simulink model "EST"  (R2022b)
settings: Solver=FixedStepAuto  StartTime=0.0  StopTime=stopt  FixedStep=deltat/10  MaxStep=0.05  RelTol=1
InitFcn:
  | clear all;
  | close all;
  | clc;
  | 
  | % add the data and script directories
  | addpath('data','scripts');
  | 
  | % load the constants (units)
  | constants;
  | 
  | % load the simulation parameters
  | preprocessing;
StopFcn:
  | postprocessing;
model workspace (MAT data in the model file):
  TDeltaStorageInitial = Simulink.Parameter
  TDeltaStorageInitial.Value = 0
  TDeltaStorageInitial.DataType = 'auto'
  TDeltaStorageInitial.Complexity = 'real'
  TDeltaStorageInitial.Dimensions = [1 1]
  TStorageMax = Simulink.Parameter
  TStorageMax.Value = 10
  TStorageMax.DataType = 'auto'
  TStorageMax.Complexity = 'real'
  TStorageMax.Dimensions = [1 1]
  TStorageMin = Simulink.Parameter
  TStorageMin.Value = 0
  TStorageMin.DataType = 'auto'
  TStorageMin.Complexity = 'real'
  TStorageMin.Dimensions = [1 1]
values from neighbouring files (symbols this model uses):
  aDemandTransport = 0.02    [preprocessing.m]
  aExtraction = 0.11    [preprocessing.m]
  aNetInjection = 0.05    [preprocessing.m]
  areaOfTank = 6096*unit("m")*unit("m")    [preprocessing.m]
  bStorage = 1e-8/unit("s")    [preprocessing.m]
  e = 0.07    [preprocessing.m]
  efficiencyInverter = 0.97    [preprocessing.m]
  efficiencyTransformer = 0.99    [preprocessing.m]
  environmentalTemperature = 293*unit("K")    [preprocessing.m]
  EStorageInitial = 0.0*unit("kWh")    [preprocessing.m]
  EStorageMax = 450000*unit("kWh")    [preprocessing.m]
  EStorageMin = 0.0*unit("kWh")    [preprocessing.m]
  k = 0.04*unit("W")/unit("m")/unit("K")    [preprocessing.m]
  mass = 25837320*unit("kg")    [preprocessing.m]
  resistance = 0.00002373556*unit("ohm")    [preprocessing.m]
  sb = 5.670374419*10^-8*(     unit("W")/unit("m")/unit("m")/unit("K")/unit("K")/unit("K")/unit("K"))    [preprocessing.m]
  stringVoltage = 408*unit("V")    [preprocessing.m]
  x = 1*unit("m")    [preprocessing.m]
settings Model: Creator=joche  LastModifiedBy=20231162
settings DataIOCC: SaveFormat=Array  SaveOutput=off  ReturnWorkspaceOutputs=off
settings DebuggingCC: UnderSpecifiedDimensionMsg=warning
settings ModelReferenceCC: EnableRefExpFcnMdlSchedulingChecks=on

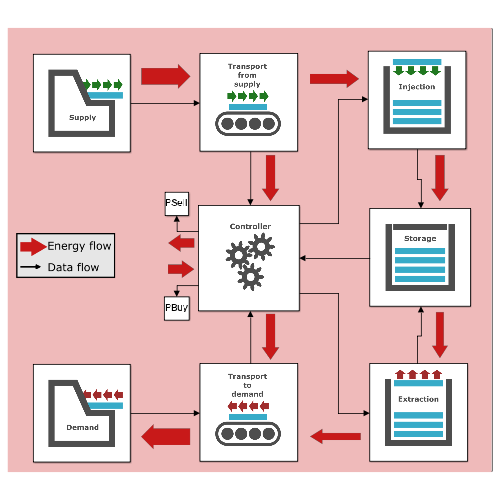
[thumbnail: Simulink's stored preview of the top-level diagram]
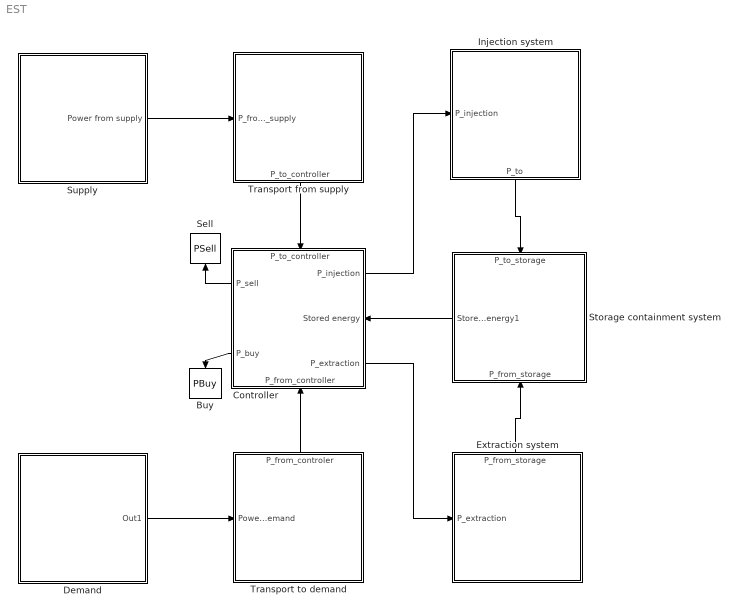
== system EST ==
  Buy : ToWorkspace  VariableName=PBuy  SampleTime=-1
  Controller : Subsystem
      settings: PortSchema="{\"entries\":[{\"content\":{\"sides\":[{\"content\":{\"connectorIds\":[\"Out3\",\"Out4\"]},\"type\":\"ConnectorPlacement.EquallySpacedRectSide\",\"uuid\":\"4daf33ce-c96a-4783-b5c4-228eed953e01\"},{\"content\":{\"connectorIds\":[\"Out1\",\"In3\",\"Out2\"],\"side\":\"RIGHT\"},\"type\":\"ConnectorPlacement.EquallySpacedRectSide\",\"uuid\":\"e9942e50-8467-4af8-b79b-80636cbc76e5\"},{\"content\":{\"connectorIds\":[\"In1\"],\"side\":\"TOP\"},\"type\":\"ConnectorPlacement.EquallySpacedRectSide\",\"uuid\":\"f315e931-d69b-4751-b712-f89c6c81baeb\"},{\"content\":{\"connectorIds\":[\"In2\"],\"side\":\"BOTTOM\"},\"type\":\"ConnectorPlacement.EquallySpacedRectSide\",\"uuid\":\"44715ee6-5cd5-4669-bcb9-5ed7c869bdb3\"}]},\"type\":\"ConnectorPlacement.EquallySpacedConnector\",\"uuid\":\"fff48899-944b-4064-b7d7-ecc12144fb48\"}],\"packageUris\":[\"http://schema.mathworks.com/mf0/Connector/R2020b\"],\"version\":\"1.0\"}"
      mask Display: image('$imagefile'); % Use "Edit Image" on toolstrip to change.
  Demand : Subsystem
      mask Display: image('$imagefile'); % Use "Edit Image" on toolstrip to change.
  Extraction system : Subsystem
      settings: PortSchema="{\"entries\":[{\"content\":{\"sides\":[{\"content\":{\"connectorIds\":[]},\"type\":\"ConnectorPlacement.EquallySpacedRectSide\",\"uuid\":\"05c5933d-55fc-4e06-853f-fc26d42905f9\"},{\"content\":{\"connectorIds\":[\"In1\"],\"side\":\"RIGHT\"},\"type\":\"ConnectorPlacement.EquallySpacedRectSide\",\"uuid\":\"327426c5-31d5-498b-a2bd-83e49353408c\"},{\"content\":{\"connectorIds\":[],\"side\":\"TOP\"},\"type\":\"ConnectorPlacement.EquallySpacedRectSide\",\"uuid\":\"55306cf3-a3de-4385-a5ae-b8600ecdd5a2\"},{\"content\":{\"connectorIds\":[\"Out1\"],\"side\":\"BOTTOM\"},\"type\":\"ConnectorPlacement.EquallySpacedRectSide\",\"uuid\":\"08fcc9c3-40d3-4ac6-b914-dfeef6039ffb\"}]},\"type\":\"ConnectorPlacement.EquallySpacedConnector\",\"uuid\":\"cb35d5ba-e8c6-462c-b7b2-fe8356d4b0a1\"}],\"packageUris\":[\"http://schema.mathworks.com/mf0/Connector/R2020b\"],\"version\":\"1.0\"}"
      mask Display: image('$imagefile'); % Use "Edit Image" on toolstrip to change.
  Injection system : Subsystem
      settings: PortSchema="{\"entries\":[{\"content\":{\"sides\":[{\"content\":{\"connectorIds\":[]},\"type\":\"ConnectorPlacement.EquallySpacedRectSide\",\"uuid\":\"05c5933d-55fc-4e06-853f-fc26d42905f9\"},{\"content\":{\"connectorIds\":[\"In1\"],\"side\":\"RIGHT\"},\"type\":\"ConnectorPlacement.EquallySpacedRectSide\",\"uuid\":\"327426c5-31d5-498b-a2bd-83e49353408c\"},{\"content\":{\"connectorIds\":[\"Out1\"],\"side\":\"TOP\"},\"type\":\"ConnectorPlacement.EquallySpacedRectSide\",\"uuid\":\"55306cf3-a3de-4385-a5ae-b8600ecdd5a2\"},{\"content\":{\"connectorIds\":[],\"side\":\"BOTTOM\"},\"type\":\"ConnectorPlacement.EquallySpacedRectSide\",\"uuid\":\"08fcc9c3-40d3-4ac6-b914-dfeef6039ffb\"}]},\"type\":\"ConnectorPlacement.EquallySpacedConnector\",\"uuid\":\"cb35d5ba-e8c6-462c-b7b2-fe8356d4b0a1\"}],\"packageUris\":[\"http://schema.mathworks.com/mf0/Connector/R2020b\"],\"version\":\"1.0\"}"
      mask Display: image('$imagefile'); % Use "Edit Image" on toolstrip to change.
  Sell : ToWorkspace  VariableName=PSell  SampleTime=-1
  Storage containment system : Subsystem
      settings: PortSchema="{\"entries\":[{\"content\":{\"sides\":[{\"content\":{\"connectorIds\":[\"Out1\"]},\"type\":\"ConnectorPlacement.EquallySpacedRectSide\",\"uuid\":\"0ba48424-33b9-4934-970f-64fe5d8b070e\"},{\"content\":{\"connectorIds\":[],\"side\":\"RIGHT\"},\"type\":\"ConnectorPlacement.EquallySpacedRectSide\",\"uuid\":\"9cde340f-8f39-4499-9a12-5e1623737660\"},{\"content\":{\"connectorIds\":[\"In1\"],\"side\":\"TOP\"},\"type\":\"ConnectorPlacement.EquallySpacedRectSide\",\"uuid\":\"2af8db04-7fd0-4902-8637-8dc00edb4598\"},{\"content\":{\"connectorIds\":[\"In2\"],\"side\":\"BOTTOM\"},\"type\":\"ConnectorPlacement.EquallySpacedRectSide\",\"uuid\":\"e21ea806-d777-41a3-a53f-556fae66854b\"}]},\"type\":\"ConnectorPlacement.EquallySpacedConnector\",\"uuid\":\"4e2ddb36-4db3-4ab4-858b-ebb8ccefeb1f\"}],\"packageUris\":[\"http://schema.mathworks.com/mf0/Connector/R2020b\"],\"version\":\"1.0\"}"
      mask Display: image('$imagefile'); % Use "Edit Image" on toolstrip to change.
  Supply : Subsystem
      mask Display: image('$imagefile'); % Use "Edit Image" on toolstrip to change.
  Transport from supply : Subsystem
      settings: PortSchema="{\"entries\":[{\"content\":{\"sides\":[{\"content\":{\"connectorIds\":[\"In1\"]},\"type\":\"ConnectorPlacement.EquallySpacedRectSide\",\"uuid\":\"31329006-3d36-4d93-9c44-7503a515d397\"},{\"content\":{\"connectorIds\":[],\"side\":\"RIGHT\"},\"type\":\"ConnectorPlacement.EquallySpacedRectSide\",\"uuid\":\"aba139c7-f9b6-4881-a56b-a4cbbedacd88\"},{\"content\":{\"connectorIds\":[],\"side\":\"TOP\"},\"type\":\"ConnectorPlacement.EquallySpacedRectSide\",\"uuid\":\"e683eb73-7a35-4160-9c39-da83856a6278\"},{\"content\":{\"connectorIds\":[\"Out1\"],\"side\":\"BOTTOM\"},\"type\":\"ConnectorPlacement.EquallySpacedRectSide\",\"uuid\":\"1170dd18-447c-437f-9043-6812c2877331\"}]},\"type\":\"ConnectorPlacement.EquallySpacedConnector\",\"uuid\":\"804af608-1d70-444f-af69-e05f19bf98f3\"}],\"packageUris\":[\"http://schema.mathworks.com/mf0/Connector/R2020b\"],\"version\":\"1.0\"}"
      mask Display: image('$imagefile'); % Use "Edit Image" on toolstrip to change.
  Transport to demand : Subsystem
      settings: PortSchema="{\"entries\":[{\"content\":{\"sides\":[{\"content\":{\"connectorIds\":[\"In1\"]},\"type\":\"ConnectorPlacement.EquallySpacedRectSide\",\"uuid\":\"31329006-3d36-4d93-9c44-7503a515d397\"},{\"content\":{\"connectorIds\":[],\"side\":\"RIGHT\"},\"type\":\"ConnectorPlacement.EquallySpacedRectSide\",\"uuid\":\"aba139c7-f9b6-4881-a56b-a4cbbedacd88\"},{\"content\":{\"connectorIds\":[\"Out1\"],\"side\":\"TOP\"},\"type\":\"ConnectorPlacement.EquallySpacedRectSide\",\"uuid\":\"e683eb73-7a35-4160-9c39-da83856a6278\"},{\"content\":{\"connectorIds\":[],\"side\":\"BOTTOM\"},\"type\":\"ConnectorPlacement.EquallySpacedRectSide\",\"uuid\":\"c378138f-7233-4483-870c-40a69b3495ee\"}]},\"type\":\"ConnectorPlacement.EquallySpacedConnector\",\"uuid\":\"804af608-1d70-444f-af69-e05f19bf98f3\"}],\"packageUris\":[\"http://schema.mathworks.com/mf0/Connector/R2020b\"],\"version\":\"1.0\"}"
      mask Display: image('$imagefile'); % Use "Edit Image" on toolstrip to change.
  wires:
  Supply/1(Power from supply) -> Transport from supply/1(P_from_supply)
  Transport from supply/1(P_to_controller) -> Controller/1(P_to_controller)
  Transport to demand/1(P_from_controler) -> Controller/2(P_from_controller)
  Demand/1(Out1) -> Transport to demand/1(Power to demand)
  Controller/3(P_sell) -> Sell/1
  Controller/2(P_extraction) -> Extraction system/1(P_extraction)
  Injection system/1(P_to) -> Storage containment system/1(P_to_storage)
  Extraction system/1(P_from_storage) -> Storage containment system/2(P_from_storage)
  Storage containment system/1(Stored energy1) -> Controller/3(Stored energy)
  Controller/1(P_injection) -> Injection system/1(P_injection)
  Controller/4(P_buy) -> Buy/1

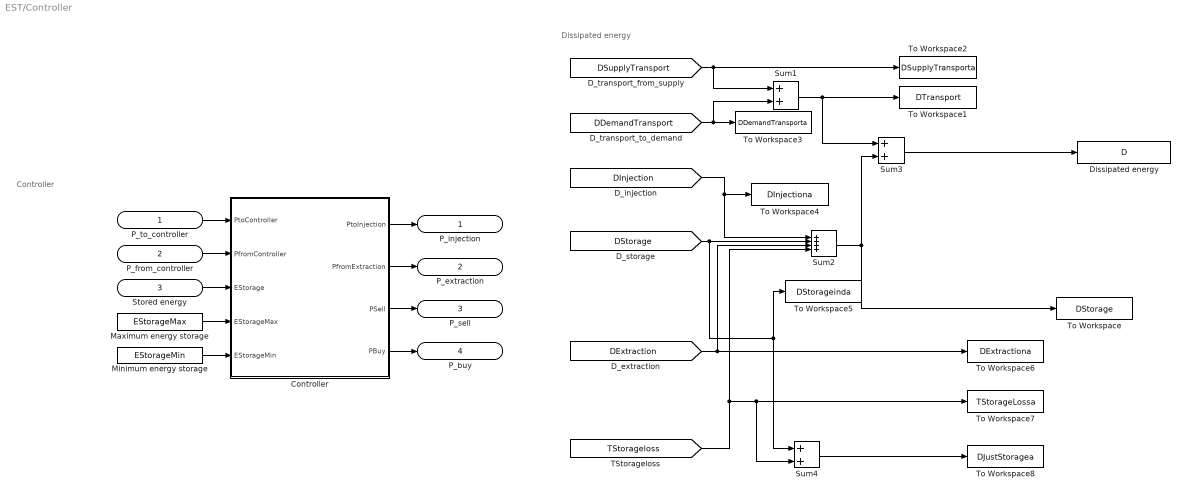
== system EST/Controller ==
  note: Dissipated energy
  note: Controller
  P_to_controller : Inport
  P_from_controller : Inport  Port=2
  Stored energy : Inport  Port=3
  Controller : MATLAB Function  TreatAsAtomicUnit=on
  Dissipated energy : ToWorkspace  VariableName=D  SampleTime=-1
  Maximum energy storage : Constant  Value=EStorageMax
  Minimum energy storage : Constant  Value=EStorageMin
  Sum1 : Sum
  Sum2 : Sum  Inputs=++++
  Sum3 : Sum
  Sum4 : Sum
  To Workspace : ToWorkspace  VariableName=DStorage  SampleTime=-1
  To Workspace1 : ToWorkspace  VariableName=DTransport  SampleTime=-1
  To Workspace2 : ToWorkspace  VariableName=DSupplyTransporta  SampleTime=-1
  To Workspace3 : ToWorkspace  VariableName=DDemandTransporta  SampleTime=-1
  To Workspace4 : ToWorkspace  VariableName=DInjectiona  SampleTime=-1
  To Workspace5 : ToWorkspace  VariableName=DStorageinda  SampleTime=-1
  To Workspace6 : ToWorkspace  VariableName=DExtractiona  SampleTime=-1
  To Workspace7 : ToWorkspace  VariableName=TStorageLossa  SampleTime=-1
  To Workspace8 : ToWorkspace  VariableName=DJustStoragea  SampleTime=-1
  P_injection : Outport
  P_extraction : Outport  Port=2
  P_sell : Outport  Port=3
  P_buy : Outport  Port=4
  wires:
  P_from_controller/1 -> Controller/2(PfromController)
  Controller/2(PfromExtraction) -> P_extraction/1
  Controller/3(PSell) -> P_sell/1
  Controller/4(PBuy) -> P_buy/1
  Minimum energy storage/1 -> Controller/5(EStorageMin)
  Maximum energy storage/1 -> Controller/4(EStorageMax)
  P_to_controller/1 -> Controller/1(PtoController)
  Controller/1(PtoInjection) -> P_injection/1
  Stored energy/1 -> Controller/3(EStorage)
  [DDemandTransport] -> Sum1/2, To Workspace3/1
  [DSupplyTransport] -> Sum1/1, To Workspace2/1
  [DInjection] -> Sum2/1, To Workspace4/1
  [DStorage] -> Sum2/2, Sum4/1, To Workspace5/1
  [DExtraction] -> Sum2/3, To Workspace6/1
  Sum2/1 -> To Workspace/1, Sum3/2
  Sum1/1 -> Sum3/1, To Workspace1/1
  Sum3/1 -> Dissipated energy/1
  [TStorageloss] -> Sum2/4, Sum4/2, To Workspace7/1
  Sum4/1 -> To Workspace8/1

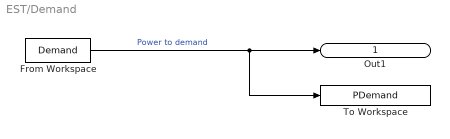
== system EST/Demand ==
  From Workspace : FromWorkspace  VariableName=Demand  OutputAfterFinalValue=Setting to zero
  To Workspace : ToWorkspace  VariableName=PDemand  SampleTime=-1
  Out1 : Outport
  wires:
  From Workspace/1 -> To Workspace/1, Out1/1  "Power to demand"

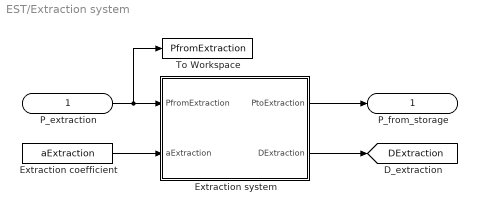
== system EST/Extraction system ==
  P_extraction : Inport
  Extraction coefficient : Constant  Value=aExtraction
  Extraction system : MATLAB Function  TreatAsAtomicUnit=on
  To Workspace : ToWorkspace  VariableName=PfromExtraction  SampleTime=-1
  P_from_storage : Outport
  tag scope: DExtraction=global
  wires:
  P_extraction/1 -> To Workspace/1, Extraction system/1(PfromExtraction)
  Extraction system/1(PtoExtraction) -> P_from_storage/1
  Extraction coefficient/1 -> Extraction system/2(aExtraction)
  Extraction system/2(DExtraction) -> [DExtraction]

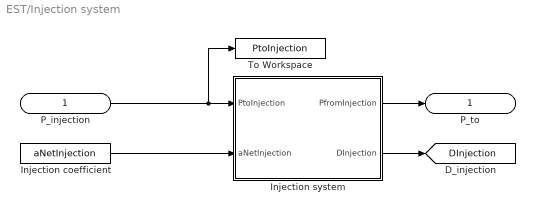
== system EST/Injection system ==
  P_injection : Inport
  Injection coefficient : Constant  Value=aNetInjection
  Injection system : MATLAB Function  TreatAsAtomicUnit=on
  To Workspace : ToWorkspace  VariableName=PtoInjection  SampleTime=-1
  P_to : Outport
  tag scope: DInjection=global
  wires:
  P_injection/1 -> To Workspace/1, Injection system/1(PtoInjection)
  Injection system/1(PfromInjection) -> P_to/1
  Injection coefficient/1 -> Injection system/2(aNetInjection)
  Injection system/2(DInjection) -> [DInjection]

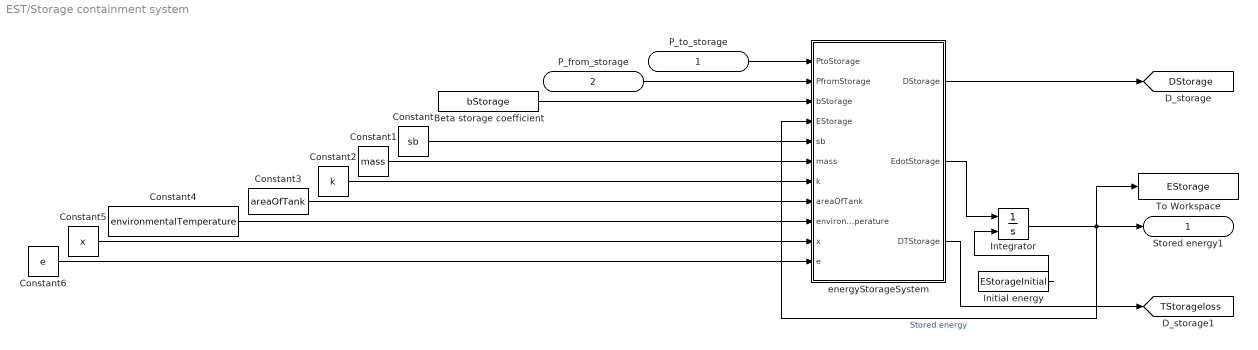
== system EST/Storage containment system ==
  P_to_storage : Inport
  P_from_storage : Inport  Port=2
  Beta storage coefficient : Constant  Value=bStorage
  Constant : Constant  Value=sb
  Constant1 : Constant  Value=mass
  Constant2 : Constant  Value=k
  Constant3 : Constant  Value=areaOfTank
  Constant4 : Constant  Value=environmentalTemperature
  Constant5 : Constant  Value=x
  Constant6 : Constant  Value=e
  Initial energy : Constant  Value=EStorageInitial
  Integrator : Integrator  InitialConditionSource=external
  To Workspace : ToWorkspace  VariableName=EStorage  SampleTime=-1
  energyStorageSystem : MATLAB Function  TreatAsAtomicUnit=on
  Stored energy1 : Outport
  tag scope: DStorage=global, TStorageloss=global
  wires:
  Initial energy/1 -> Integrator/2
  Integrator/1 -> To Workspace/1, energyStorageSystem/4(EStorage), Stored energy1/1  "Stored energy"
  energyStorageSystem/1(DStorage) -> [DStorage]
  Beta storage coefficient/1 -> energyStorageSystem/3(bStorage)
  energyStorageSystem/2(EdotStorage) -> Integrator/1
  P_to_storage/1 -> energyStorageSystem/1(PtoStorage)
  P_from_storage/1 -> energyStorageSystem/2(PfromStorage)
  energyStorageSystem/3(DTStorage) -> [TStorageloss]
  Constant/1 -> energyStorageSystem/5(sb)
  Constant1/1 -> energyStorageSystem/6(mass)
  Constant2/1 -> energyStorageSystem/7(k)
  Constant3/1 -> energyStorageSystem/8(areaOfTank)
  Constant4/1 -> energyStorageSystem/9(environmentalTemperature)
  Constant5/1 -> energyStorageSystem/10(x)
  Constant6/1 -> energyStorageSystem/11(e)

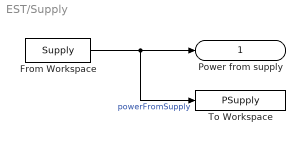
== system EST/Supply ==
  From Workspace : FromWorkspace  VariableName=Supply  OutputAfterFinalValue=Setting to zero
  To Workspace : ToWorkspace  VariableName=PSupply  SampleTime=-1
  Power from supply : Outport
  wires:
  From Workspace/1 -> To Workspace/1, Power from supply/1  "powerFromSupply"

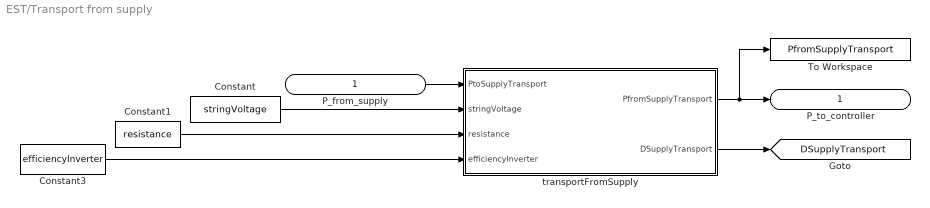
== system EST/Transport from supply ==
  P_from_supply : Inport
  " transportFromSupply" : MATLAB Function  TreatAsAtomicUnit=on
  Constant : Constant  Value=stringVoltage
  Constant1 : Constant  Value=resistance
  Constant3 : Constant  Value=efficiencyInverter
  To Workspace : ToWorkspace  VariableName=PfromSupplyTransport  SampleTime=-1
  P_to_controller : Outport
  tag scope: DSupplyTransport=global
  wires:
  P_from_supply/1 -> " transportFromSupply"/1(PtoSupplyTransport)
  " transportFromSupply"/1(PfromSupplyTransport) -> To Workspace/1, P_to_controller/1
  " transportFromSupply"/2(DSupplyTransport) -> [DSupplyTransport]
  Constant/1 -> " transportFromSupply"/2(stringVoltage)
  Constant1/1 -> " transportFromSupply"/3(resistance)
  Constant3/1 -> " transportFromSupply"/4(efficiencyInverter)

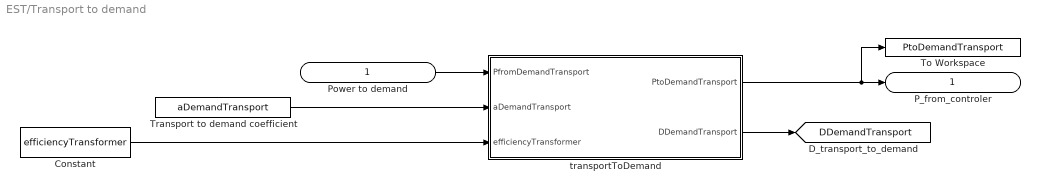
== system EST/Transport to demand ==
  Power to demand : Inport
  Constant : Constant  Value=efficiencyTransformer
  To Workspace : ToWorkspace  VariableName=PtoDemandTransport  SampleTime=-1
  Transport to demand coefficient : Constant  Value=aDemandTransport
  transportToDemand : MATLAB Function  TreatAsAtomicUnit=on
  P_from_controler : Outport
  tag scope: DDemandTransport=global
  wires:
  Transport to demand coefficient/1 -> transportToDemand/2(aDemandTransport)
  transportToDemand/2(DDemandTransport) -> [DDemandTransport]
  transportToDemand/1(PtoDemandTransport) -> To Workspace/1, P_from_controler/1
  Power to demand/1 -> transportToDemand/1(PfromDemandTransport)
  Constant/1 -> transportToDemand/3(efficiencyTransformer)

== matlab function EST/Injection system/Injection system ==
  data: PtoInjection input; PfromInjection output; aNetInjection input; DInjection output
function [PfromInjection, DInjection] = injection(PtoInjection, aNetInjection ...
    )
    %
    % This function calculates the power signal and coreresponding loss 
    % after the injection. The returned power signal goes to the air energy
    % storage as well as the thermal storage.
    %
    % Parameters:
    %   PtoInjection: A double with the power signals coming from the
    %                 supply required by the controller with the same array 
    %                 dimensions as tout.
    %   aInjection:   A double of size 1x1 which is the loss coeficient
    %                 during injection.
    %
    % Returns:
    %   double: PfromInjection, the power signal with the same
    %           array dimensions as PtoInjection. Goes to the storage.
    %   double: DInjection, the dissipation signal with the same
    %           array dimensions as PtoInjection.

    % Find the dissipation by multiplying the loss coefficent by the power
    % signal.
    DInjection = aNetInjection*PtoInjection;
    % Calculate the power signal that goes to the storage by subtracting
    % the dissipation from the original power signal.
    PfromInjection = PtoInjection - DInjection;
end

== matlab function EST/Transport from supply/ transportFromSupply ==
  data: PtoSupplyTransport input; PfromSupplyTransport output; DSupplyTransport output; stringVoltage input; resistance input; efficiencyInverter input
function [PfromSupplyTransport, DSupplyTransport] = supplyTransport(...
    PtoSupplyTransport, stringVoltage, resistance, efficiencyInverter)
    %
    % This function calculates the power signal and coreresponding loss 
    % after the transport from the solar panels to the storage.
    %
    % Parameters:
    %   PtoSupplyTransport: A double with the power signals coming from the
    %                       supply with the same array dimensions as tout.
    %
    % Returns:
    %   double: PfromSupplyTransport, the power signal with the same
    %           array dimensions as tout.
    %   double: DSupplyTransport, the power loss signal with the same
    %           array dimensions as tout.
    %

    % Find the current in the wires in the solar panel strings before the
    % inverter.
    % Use I = P/V
    current = PtoSupplyTransport/stringVoltage;
    % Find the power loss in the wires by multiplying the square of the
    % current of one string by the amount of strings and the resistance of
    % each wire, considering that the distance from each string to the
    % converter is equal. 
    % Use P_Loss = ammountOfWires*I^2*R.
    powerLossTransport = 171*(current^2)*resistance;
    % Before the converter converts the power signals, the loss is
    % subtracted from the power from the supply so that the model can use
    % this new array.
    powerBeforeInverter = PtoSupplyTransport - powerLossTransport;
    % Assume that the inverter that converts the direct current, DC, to
    % alternating current, AC, has an efficiency of 97 percent which is 
    % quite high.
    DSupplyTransport = powerBeforeInverter*(1 - efficiencyInverter) ...
        + powerLossTransport;
    PfromSupplyTransport = (... 
        PtoSupplyTransport - DSupplyTransport + powerLossTransport);

== matlab function EST/Controller/Controller ==
  data: PtoInjection output; PfromExtraction output; PSell output; PBuy output; PtoController input; PfromController input; EStorage input; EStorageMax input; EStorageMin input
function [PtoInjection, PfromExtraction, PSell, PBuy] = controller(PtoController, PfromController, EStorage, EStorageMax, EStorageMin)
    
    %% Power surplus or deficit

    deltaP = PtoController - PfromController;

    % Power surplus
    if deltaP >= 0

        %% Storage injection

        % Storage system is not full
        if (EStorage < EStorageMax)
            PtoInjection = deltaP;

        % Storage system is full
        else
            PtoInjection = 0;
        end

        %% Storage extraction

        PfromExtraction = 0;

        %% Load-balancing
        PSell   = deltaP - PtoInjection;
        PBuy    = 0;

    % Power deficit
    else

        %% Storage injection

        PtoInjection = 0;

        %% Storage extraction

        % Storage system is not empty
        if (EStorage > EStorageMin)
            PfromExtraction = -deltaP;

        % Storage system is empty
        else
            PfromExtraction = 0;
        end

        %% Load-balancing

        PSell = 0;
        PBuy  = -deltaP - PfromExtraction;
    end

== matlab function EST/Extraction system/Extraction system ==
  data: PfromExtraction input; PtoExtraction output; aExtraction input; DExtraction output
function [PtoExtraction, DExtraction] = extraction(...
    PfromExtraction, aExtraction)
    %
    % This function calculates the power signal and coreresponding loss 
    % after the extraction. The returned power signal goes to the demand.
    %
    % Parameters:
    %   PfromExtraction: A double with the power signals that must go to
    %                    the demand as required by the controller, from
    %                    storage with the same array dimensions as tout.
    %   aExtraction:     A double of the size 1x1, which is the extraction
    %                    coefficient that can be used to calculate energy
    %                    losses during generation.
    %
    % Returns:
    %   double: PtoExtraction, the power signal with the same
    %           array dimensions as PtoInjection. Goes to demand.
    %   double: DExtraction, the dissipation signal with the same
    %           array dimensions as PfromExtraction.

    % Find the dissipation by multiplying the loss coefficent by the power
    % signal.
    DExtraction = aExtraction*PfromExtraction;
    % Calculate the power signal that goes to the demand by subtracting
    % the dissipation from the original power signal.
    PtoExtraction = PfromExtraction - DExtraction;
end

== matlab function EST/Storage containment system/energyStorageSystem ==
  data: DStorage output; EdotStorage output; PtoStorage input; PfromStorage input; bStorage input; EStorage input; DTStorage output; sb input; mass input; k input; areaOfTank input; environmentalTemperature input; x input; e input
function [DStorage, EdotStorage, DTStorage]= Storage(...
    PtoStorage, PfromStorage, bStorage, EStorage, sb, mass, k, ...
    areaOfTank, environmentalTemperature, x, e)
    %
    % This function calculates the change in the energy storage of both the
    % air storage and thermal storage. To do this the dissipations are also
    % calculated. It is assumed that one quarter of the energy is stored in 
    % the thermal storage.
    %
    % Parameters:
    %   PtoStorage:   A double with the power signals coming from the
    %                 supply required by the controller with the same array 
    %                 dimensions as tout.
    %   PfromStorage: A double with the power signals heading to the
    %                 extraction required by the controller with the same
    %                 array dimensions as tout.
    %   bStorage:     A double of size 1x1, which is used to calculate the
    %                 dissipation of the energy storage.
    %   EStorage:     A double with the energy values for the energy
    %                 storage with the same array dimensions as tout.
    %
    % Returns:
    %   double: DStorage, the dissipation signal for the air storage with 
    %           the same array dimensions as PtoStorage.
    %   double: EdotStorage, the change in energy stored per time unit, 
    %           with the same array dimensions as PtoStorage.
    %   double: DTStorage, the dissipation signal for the thermal storage
    %           with the same array dimensions as PtoStorage.
    %

    % The dissipation of the air storage can be calculated by
    % multiplying the storage loss coefficent by the amount of energy
    % stored in the air storage which is three quarters of the total
    % energy.
    DStorage = bStorage*(0.75*EStorage);

    % The temperature of the thermal storage is calculated based on the
    % stored energy and the parameters of the thermal storage.
    T = 0.25*EStorage/(mass*4180) + environmentalTemperature; % Temperature
    % The dissipation of the thermal storage is based on conduction and 
    % radiation.
    DTStorage = k*areaOfTank*(T-environmentalTemperature)/x + (...
        sb*e*areaOfTank*(T^4 - environmentalTemperature^4));
    EdotStorage = 0.75*PtoStorage - 0.75*PfromStorage - DStorage + (... 
        0.25*PtoStorage - 0.25*PfromStorage) - DTStorage;

== matlab function EST/Transport to demand/transportToDemand ==
  data: PfromDemandTransport input; PtoDemandTransport output; aDemandTransport input; DDemandTransport output; efficiencyTransformer input
function [PtoDemandTransport, DDemandTransport] = demandTransport(... 
    PfromDemandTransport, aDemandTransport, efficiencyTransformer)
    %
    % This function calculates the power signal and coreresponding loss 
    % after the extraction. The returned power signal goes to the demand.
    %
    % Parameters:
    %   PfromDemandTransport:  A double with the power signals that must go
    %                          to the demand as required by the controller,
    %                          from storage with the same array dimensions 
    %                          as tout.
    %   aDemandTransport:      A double of the size 1x1, which is the
    %                          transport coefficient that can be used to
    %                          calculate energy losses during transport.
    %
    % Returns:
    %   double: PtoDemandTransport, the power signal with the same
    %           array dimensions as PfromDemandTransport.
    %   double: DDemandTransport, the dissipation signal with the same
    %           array dimensions as PfromDemandTransport.

    % Before this there is the step-up transformer which has a loss of one 
    % percent.
    % Roughly two percent lost over a length of 60 kilometers.
    DDemandTransport = (aDemandTransport + (1 - efficiencyTransformer) ... 
        + (1 - efficiencyTransformer))*PfromDemandTransport;
    % Subtract the power loss from the power signal to find the final
    % signal delivered to the building in Amsterdam.
    PtoDemandTransport = PfromDemandTransport - DDemandTransport;
    % After this there is a step-down transformer.
end
